simulink model "test_mdl_NI"  (R2018a)
settings: Solver=VariableStepAuto  StartTime=0.0  StopTime=10.0  RelTol=1e-3
(part 8 of 24)

== system test_mdl_NI/Subsystem/ECM_Diesel/Powertrain_Data_4_Ox424 ==
  in_port : Inport
  BpedDrvMsgTxt_B_Dsply : Terminator
  FuelLvlWarn_D_ActlEng : Terminator
  FuelLvl_Pc_DsplyEng : Terminator
  FuelRange_L_DsplyEng : Terminator
  RearDiffOilTeWarn_B_Rq : Terminator
  RearDiffOil_Te_Actl : Terminator
  SelDrvMdePt_D_Stat : Terminator
  bus_selector : BusSelector  OutputSignals=BpedDrvMsgTxt_B_Dsply,FuelLvlWarn_D_ActlEng,FuelLvl_Pc_DsplyEng,FuelRange_L_DsplyEng,RearDiffOilTeWarn_B_Rq,RearDiffOil_Te_Actl,SelDrvMdePt_D_Stat
  wires:
  in_port/1 -> bus_selector/1  "Powertrain_Data_4_Ox424"
  bus_selector/1 -> BpedDrvMsgTxt_B_Dsply/1  "<BpedDrvMsgTxt_B_Dsply>"
  bus_selector/2 -> FuelLvlWarn_D_ActlEng/1  "<FuelLvlWarn_D_ActlEng>"
  bus_selector/3 -> FuelLvl_Pc_DsplyEng/1  "<FuelLvl_Pc_DsplyEng>"
  bus_selector/4 -> FuelRange_L_DsplyEng/1  "<FuelRange_L_DsplyEng>"
  bus_selector/5 -> RearDiffOilTeWarn_B_Rq/1  "<RearDiffOilTeWarn_B_Rq>"
  bus_selector/6 -> RearDiffOil_Te_Actl/1  "<RearDiffOil_Te_Actl>"
  bus_selector/7 -> SelDrvMdePt_D_Stat/1  "<SelDrvMdePt_D_Stat>"

== system test_mdl_NI/Subsystem/ECM_Diesel/Powertrain_Data_5_Ox43F ==
  in_port : Inport
  AdasLcObtclAbrt_B_Stat : Terminator
  AirDamPos_D_Stat : Terminator
  BattRgenLoChrg_D_RqEng : Terminator
  BattRgenLoDChrg_D_RqEng : Terminator
  FapLcActv_B_Stat : Terminator
  FapLcInhbt_B_Rq : Terminator
  FapLcMaxGrdAbrt_B_Stat : Terminator
  FapLcMaxGrdInhbt_B_Stat : Terminator
  FapLcObstcl_B_Stat : Terminator
  FapLcPrchgBrk_B_Rq : Terminator
  FapLcStopHold_B_Rq : Terminator
  bus_selector : BusSelector  OutputSignals=AdasLcObtclAbrt_B_Stat,AirDamPos_D_Stat,BattRgenLoChrg_D_RqEng,BattRgenLoDChrg_D_RqEng,FapLcActv_B_Stat,FapLcInhbt_B_Rq,FapLcMaxGrdAbrt_B_Stat,FapLcMaxGrdInhbt_B_Stat,FapLcObstcl_B_Stat,FapLcPrchgBrk_B_Rq,FapLcStopHold_B_Rq
  wires:
  in_port/1 -> bus_selector/1  "Powertrain_Data_5_Ox43F"
  bus_selector/1 -> AdasLcObtclAbrt_B_Stat/1  "<AdasLcObtclAbrt_B_Stat>"
  bus_selector/2 -> AirDamPos_D_Stat/1  "<AirDamPos_D_Stat>"
  bus_selector/3 -> BattRgenLoChrg_D_RqEng/1  "<BattRgenLoChrg_D_RqEng>"
  bus_selector/4 -> BattRgenLoDChrg_D_RqEng/1  "<BattRgenLoDChrg_D_RqEng>"
  bus_selector/5 -> FapLcActv_B_Stat/1  "<FapLcActv_B_Stat>"
  bus_selector/6 -> FapLcInhbt_B_Rq/1  "<FapLcInhbt_B_Rq>"
  bus_selector/7 -> FapLcMaxGrdAbrt_B_Stat/1  "<FapLcMaxGrdAbrt_B_Stat>"
  bus_selector/8 -> FapLcMaxGrdInhbt_B_Stat/1  "<FapLcMaxGrdInhbt_B_Stat>"
  bus_selector/9 -> FapLcObstcl_B_Stat/1  "<FapLcObstcl_B_Stat>"
  bus_selector/10 -> FapLcPrchgBrk_B_Rq/1  "<FapLcPrchgBrk_B_Rq>"
  bus_selector/11 -> FapLcStopHold_B_Rq/1  "<FapLcStopHold_B_Rq>"

== system test_mdl_NI/Subsystem/ECM_Diesel/Stop_Start_Ox166 ==
  in_port : Inport
  AutoStopPtDelta_I_Est : Terminator
  HiElPwInhbt_B_Stat : Terminator
  OdoTripVerify_L_Actl : Terminator
  StopStrtDrvMde_D_Indic : Terminator
  StopStrtIODTxt_D_Rq : Terminator
  StopStrtMsgTxt_D_Rq : Terminator
  StopStrtStdby_D_Indic : Terminator
  bus_selector : BusSelector  OutputSignals=AutoStopPtDelta_I_Est,HiElPwInhbt_B_Stat,OdoTripVerify_L_Actl,StopStrtDrvMde_D_Indic,StopStrtIODTxt_D_Rq,StopStrtMsgTxt_D_Rq,StopStrtStdby_D_Indic
  wires:
  in_port/1 -> bus_selector/1  "Stop_Start_Ox166"
  bus_selector/1 -> AutoStopPtDelta_I_Est/1  "<AutoStopPtDelta_I_Est>"
  bus_selector/2 -> HiElPwInhbt_B_Stat/1  "<HiElPwInhbt_B_Stat>"
  bus_selector/3 -> OdoTripVerify_L_Actl/1  "<OdoTripVerify_L_Actl>"
  bus_selector/4 -> StopStrtDrvMde_D_Indic/1  "<StopStrtDrvMde_D_Indic>"
  bus_selector/5 -> StopStrtIODTxt_D_Rq/1  "<StopStrtIODTxt_D_Rq>"
  bus_selector/6 -> StopStrtMsgTxt_D_Rq/1  "<StopStrtMsgTxt_D_Rq>"
  bus_selector/7 -> StopStrtStdby_D_Indic/1  "<StopStrtStdby_D_Indic>"

== system test_mdl_NI/Subsystem/ECM_Diesel/TesterPhysicalResPCM_Ox7E8 ==
  in_port : Inport
  TesterPhysicalResPCM : Terminator
  bus_selector : BusSelector  OutputSignals=TesterPhysicalResPCM
  wires:
  in_port/1 -> bus_selector/1  "TesterPhysicalResPCM_Ox7E8"
  bus_selector/1 -> TesterPhysicalResPCM/1  "<TesterPhysicalResPCM>"

== system test_mdl_NI/Subsystem/ECM_Diesel/TesterPhysicalResSOBDMCFD1_Ox7EE ==
  in_port : Inport
  TesterPhysicalResSOBDMC : Terminator
  bus_selector : BusSelector  OutputSignals=TesterPhysicalResSOBDMC
  wires:
  in_port/1 -> bus_selector/1  "TesterPhysicalResSOBDMCFD1_Ox7EE"
  bus_selector/1 -> TesterPhysicalResSOBDMC/1  "<TesterPhysicalResSOBDMC>"

== system test_mdl_NI/Subsystem/ECM_Diesel/TorqueDataEngFlags_Ox200 ==
  in_port : Inport
  PrplWhlTotTqRq_No_Cnt : Terminator
  PrplWhlTotTqRq_No_Cs : Terminator
  PrplWhlTot_Tq_LimMn : Terminator
  PrplWhlTot_Tq_Rq : Terminator
  PtDrvMde_D_Stat : Terminator
  bus_selector : BusSelector  OutputSignals=PrplWhlTotTqRq_No_Cnt,PrplWhlTotTqRq_No_Cs,PrplWhlTot_Tq_LimMn,PrplWhlTot_Tq_Rq,PtDrvMde_D_Stat
  wires:
  in_port/1 -> bus_selector/1  "TorqueDataEngFlags_Ox200"
  bus_selector/1 -> PrplWhlTotTqRq_No_Cnt/1  "<PrplWhlTotTqRq_No_Cnt>"
  bus_selector/2 -> PrplWhlTotTqRq_No_Cs/1  "<PrplWhlTotTqRq_No_Cs>"
  bus_selector/3 -> PrplWhlTot_Tq_LimMn/1  "<PrplWhlTot_Tq_LimMn>"
  bus_selector/4 -> PrplWhlTot_Tq_Rq/1  "<PrplWhlTot_Tq_Rq>"
  bus_selector/5 -> PtDrvMde_D_Stat/1  "<PtDrvMde_D_Stat>"

== system test_mdl_NI/Subsystem/ECM_Diesel/VehicleOperatingModes_Ox167 ==
  in_port : Inport
  ElPw_D_Stat : Terminator
  ElPw_D_StatStrtStop : Terminator
  Eng_D_Stat : Terminator
  PlgActvArb_B_Actl : Terminator
  PrplWhlRgenMn_Tq_Actl : Terminator
  PrplWhlTot2_Tq_Actl : Terminator
  PwPckTq_D_Stat : Terminator
  TrnAinTq_D_Qf : Terminator
  TrnAin_Tq_Actl : Terminator
  bus_selector : BusSelector  OutputSignals=ElPw_D_Stat,ElPw_D_StatStrtStop,Eng_D_Stat,PlgActvArb_B_Actl,PrplWhlRgenMn_Tq_Actl,PrplWhlTot2_Tq_Actl,PwPckTq_D_Stat,TrnAinTq_D_Qf,TrnAin_Tq_Actl
  wires:
  in_port/1 -> bus_selector/1  "VehicleOperatingModes_Ox167"
  bus_selector/1 -> ElPw_D_Stat/1  "<ElPw_D_Stat>"
  bus_selector/2 -> ElPw_D_StatStrtStop/1  "<ElPw_D_StatStrtStop>"
  bus_selector/3 -> Eng_D_Stat/1  "<Eng_D_Stat>"
  bus_selector/4 -> PlgActvArb_B_Actl/1  "<PlgActvArb_B_Actl>"
  bus_selector/5 -> PrplWhlRgenMn_Tq_Actl/1  "<PrplWhlRgenMn_Tq_Actl>"
  bus_selector/6 -> PrplWhlTot2_Tq_Actl/1  "<PrplWhlTot2_Tq_Actl>"
  bus_selector/7 -> PwPckTq_D_Stat/1  "<PwPckTq_D_Stat>"
  bus_selector/8 -> TrnAinTq_D_Qf/1  "<TrnAinTq_D_Qf>"
  bus_selector/9 -> TrnAin_Tq_Actl/1  "<TrnAin_Tq_Actl>"

== system test_mdl_NI/Subsystem/GWM/AC_Compressor_Data_FD1_Ox411 ==
  in_port : Inport
  ElCmprBattSysU_D_Falt : Terminator
  ElCmprBattURng_D_Falt : Terminator
  ElCmprInnrErr_D_Falt : Terminator
  ElCmprLostComm_D_Falt : Terminator
  ElCmprOverLoad_D_Falt : Terminator
  ElCmprOverTe_D_Falt : Terminator
  ElCmprOverTe_D_Stat : Terminator
  ElCmprPerfErr_D_Falt : Terminator
  ElCmprSysU_D_Falt : Terminator
  ElCmprUHi_D_Stat : Terminator
  ElCmprUHi_U_Actl : Terminator
  ElCmpr_D_Stat : Terminator
  ElCmpr_N_Actl : Terminator
  ElCmpr_Pw_Actl : Terminator
  bus_selector : BusSelector  OutputSignals=ElCmprBattSysU_D_Falt,ElCmprBattURng_D_Falt,ElCmprInnrErr_D_Falt,ElCmprLostComm_D_Falt,ElCmprOverLoad_D_Falt,ElCmprOverTe_D_Falt,ElCmprOverTe_D_Stat,ElCmprPerfErr_D_Falt,ElCmprSysU_D_Falt,ElCmprUHi_D_Stat,ElCmprUHi_U_Actl,ElCmpr_D_Stat,ElCmpr_N_Actl,ElCmpr_Pw_Actl
  wires:
  in_port/1 -> bus_selector/1  "AC_Compressor_Data_FD1_Ox411"
  bus_selector/1 -> ElCmprBattSysU_D_Falt/1  "<ElCmprBattSysU_D_Falt>"
  bus_selector/2 -> ElCmprBattURng_D_Falt/1  "<ElCmprBattURng_D_Falt>"
  bus_selector/3 -> ElCmprInnrErr_D_Falt/1  "<ElCmprInnrErr_D_Falt>"
  bus_selector/4 -> ElCmprLostComm_D_Falt/1  "<ElCmprLostComm_D_Falt>"
  bus_selector/5 -> ElCmprOverLoad_D_Falt/1  "<ElCmprOverLoad_D_Falt>"
  bus_selector/6 -> ElCmprOverTe_D_Falt/1  "<ElCmprOverTe_D_Falt>"
  bus_selector/7 -> ElCmprOverTe_D_Stat/1  "<ElCmprOverTe_D_Stat>"
  bus_selector/8 -> ElCmprPerfErr_D_Falt/1  "<ElCmprPerfErr_D_Falt>"
  bus_selector/9 -> ElCmprSysU_D_Falt/1  "<ElCmprSysU_D_Falt>"
  bus_selector/10 -> ElCmprUHi_D_Stat/1  "<ElCmprUHi_D_Stat>"
  bus_selector/11 -> ElCmprUHi_U_Actl/1  "<ElCmprUHi_U_Actl>"
  bus_selector/12 -> ElCmpr_D_Stat/1  "<ElCmpr_D_Stat>"
  bus_selector/13 -> ElCmpr_N_Actl/1  "<ElCmpr_N_Actl>"
  bus_selector/14 -> ElCmpr_Pw_Actl/1  "<ElCmpr_Pw_Actl>"

== system test_mdl_NI/Subsystem/GWM/APIMGPS_Data_Nav_1_FD1_Ox462 ==
  in_port : Inport
  GPS_Latitude_Degrees : Terminator
  GPS_Latitude_Min_dec : Terminator
  GPS_Latitude_Minutes : Terminator
  GPS_Longitude_Degrees : Terminator
  GPS_Longitude_Min_dec : Terminator
  GPS_Longitude_Minutes : Terminator
  GpsHsphLattSth_D_Actl : Terminator
  GpsHsphLongEast_D_Actl : Terminator
  bus_selector : BusSelector  OutputSignals=GPS_Latitude_Degrees,GPS_Latitude_Min_dec,GPS_Latitude_Minutes,GPS_Longitude_Degrees,GPS_Longitude_Min_dec,GPS_Longitude_Minutes,GpsHsphLattSth_D_Actl,GpsHsphLongEast_D_Actl
  wires:
  in_port/1 -> bus_selector/1  "APIMGPS_Data_Nav_1_FD1_Ox462"
  bus_selector/1 -> GPS_Latitude_Degrees/1  "<GPS_Latitude_Degrees>"
  bus_selector/2 -> GPS_Latitude_Min_dec/1  "<GPS_Latitude_Min_dec>"
  bus_selector/3 -> GPS_Latitude_Minutes/1  "<GPS_Latitude_Minutes>"
  bus_selector/4 -> GPS_Longitude_Degrees/1  "<GPS_Longitude_Degrees>"
  bus_selector/5 -> GPS_Longitude_Min_dec/1  "<GPS_Longitude_Min_dec>"
  bus_selector/6 -> GPS_Longitude_Minutes/1  "<GPS_Longitude_Minutes>"
  bus_selector/7 -> GpsHsphLattSth_D_Actl/1  "<GpsHsphLattSth_D_Actl>"
  bus_selector/8 -> GpsHsphLongEast_D_Actl/1  "<GpsHsphLongEast_D_Actl>"

== system test_mdl_NI/Subsystem/GWM/APIMGPS_Data_Nav_2_FD1_Ox463 ==
  in_port : Inport
  GPS_Actual_vs_Infer_pos : Terminator
  GPS_Compass_direction : Terminator
  GPS_Pdop : Terminator
  GPS_UTC_hours : Terminator
  GPS_UTC_minutes : Terminator
  GPS_UTC_seconds : Terminator
  GpsUtcDay_No_Actl : Terminator
  GpsUtcMnth_No_Actl : Terminator
  GpsUtcYr_No_Actl : Terminator
  Gps_B_Falt : Terminator
  bus_selector : BusSelector  OutputSignals=GPS_Actual_vs_Infer_pos,GPS_Compass_direction,GPS_Pdop,GPS_UTC_hours,GPS_UTC_minutes,GPS_UTC_seconds,GpsUtcDay_No_Actl,GpsUtcMnth_No_Actl,GpsUtcYr_No_Actl,Gps_B_Falt
  wires:
  in_port/1 -> bus_selector/1  "APIMGPS_Data_Nav_2_FD1_Ox463"
  bus_selector/1 -> GPS_Actual_vs_Infer_pos/1  "<GPS_Actual_vs_Infer_pos>"
  bus_selector/2 -> GPS_Compass_direction/1  "<GPS_Compass_direction>"
  bus_selector/3 -> GPS_Pdop/1  "<GPS_Pdop>"
  bus_selector/4 -> GPS_UTC_hours/1  "<GPS_UTC_hours>"
  bus_selector/5 -> GPS_UTC_minutes/1  "<GPS_UTC_minutes>"
  bus_selector/6 -> GPS_UTC_seconds/1  "<GPS_UTC_seconds>"
  bus_selector/7 -> GpsUtcDay_No_Actl/1  "<GpsUtcDay_No_Actl>"
  bus_selector/8 -> GpsUtcMnth_No_Actl/1  "<GpsUtcMnth_No_Actl>"
  bus_selector/9 -> GpsUtcYr_No_Actl/1  "<GpsUtcYr_No_Actl>"
  bus_selector/10 -> Gps_B_Falt/1  "<Gps_B_Falt>"

== system test_mdl_NI/Subsystem/GWM/APIMGPS_Data_Nav_3_FD1_Ox464 ==
  in_port : Inport
  GPS_Hdop : Terminator
  GPS_Heading : Terminator
  GPS_MSL_altitude : Terminator
  GPS_Sat_num_in_view : Terminator
  GPS_Speed : Terminator
  GPS_Vdop : Terminator
  GPS_dimension : Terminator
  bus_selector : BusSelector  OutputSignals=GPS_Hdop,GPS_Heading,GPS_MSL_altitude,GPS_Sat_num_in_view,GPS_Speed,GPS_Vdop,GPS_dimension
  wires:
  in_port/1 -> bus_selector/1  "APIMGPS_Data_Nav_3_FD1_Ox464"
  bus_selector/1 -> GPS_Hdop/1  "<GPS_Hdop>"
  bus_selector/2 -> GPS_Heading/1  "<GPS_Heading>"
  bus_selector/3 -> GPS_MSL_altitude/1  "<GPS_MSL_altitude>"
  bus_selector/4 -> GPS_Sat_num_in_view/1  "<GPS_Sat_num_in_view>"
  bus_selector/5 -> GPS_Speed/1  "<GPS_Speed>"
  bus_selector/6 -> GPS_Vdop/1  "<GPS_Vdop>"
  bus_selector/7 -> GPS_dimension/1  "<GPS_dimension>"

== system test_mdl_NI/Subsystem/GWM/APIM_Data_FD1_Ox32B ==
  in_port : Inport
  AutoLghtOvrrd_B_RqDrv : Terminator
  DistToStopover_L_Actl : Terminator
  ExtLghtDsply_D_Stat : Terminator
  ExtLghtFront_D_RqMnu : Terminator
  ExtLghtLeft_D_RqMnu : Terminator
  ExtLghtRear_D_RqMnu : Terminator
  ExtLghtRight_D_RqMnu : Terminator
  GoTEditHr_T_RqMnu : Terminator
  GoTEditMnte_T_RqMnu : Terminator
  StopoverType_D_Stat : Terminator
  bus_selector : BusSelector  OutputSignals=AutoLghtOvrrd_B_RqDrv,DistToStopover_L_Actl,ExtLghtDsply_D_Stat,ExtLghtFront_D_RqMnu,ExtLghtLeft_D_RqMnu,ExtLghtRear_D_RqMnu,ExtLghtRight_D_RqMnu,GoTEditHr_T_RqMnu,GoTEditMnte_T_RqMnu,StopoverType_D_Stat
  wires:
  in_port/1 -> bus_selector/1  "APIM_Data_FD1_Ox32B"
  bus_selector/1 -> AutoLghtOvrrd_B_RqDrv/1  "<AutoLghtOvrrd_B_RqDrv>"
  bus_selector/2 -> DistToStopover_L_Actl/1  "<DistToStopover_L_Actl>"
  bus_selector/3 -> ExtLghtDsply_D_Stat/1  "<ExtLghtDsply_D_Stat>"
  bus_selector/4 -> ExtLghtFront_D_RqMnu/1  "<ExtLghtFront_D_RqMnu>"
  bus_selector/5 -> ExtLghtLeft_D_RqMnu/1  "<ExtLghtLeft_D_RqMnu>"
  bus_selector/6 -> ExtLghtRear_D_RqMnu/1  "<ExtLghtRear_D_RqMnu>"
  bus_selector/7 -> ExtLghtRight_D_RqMnu/1  "<ExtLghtRight_D_RqMnu>"
  bus_selector/8 -> GoTEditHr_T_RqMnu/1  "<GoTEditHr_T_RqMnu>"
  bus_selector/9 -> GoTEditMnte_T_RqMnu/1  "<GoTEditMnte_T_RqMnu>"
  bus_selector/10 -> StopoverType_D_Stat/1  "<StopoverType_D_Stat>"

== system test_mdl_NI/Subsystem/GWM/APIM_Request_Signals_1_FD1_Ox227 ==
  in_port : Inport
  Btt_L_Actl2 : Terminator
  ChrgCrdLckEnbl_B_Stat : Terminator
  ChrgOvrdExitScrn_D_Rq : Terminator
  Cntr_Plg_Mode_Cmd : Terminator
  EmPrflButtnAssoc_D_Rq : Terminator
  EmPrflKeyAssoc_D_Rq : Terminator
  EmPrflNo_D_Rq : Terminator
  Em_D_Stat : Terminator
  PmCabnLvl_D_Stat : Terminator
  PmCabn_D_Stat : Terminator
  PwRnngBoardMde_D_Rq : Terminator
  PwRnngBoardSwtch_D_Rq : Terminator
  PwRnngBoardT_D_Rq : Terminator
  Rba_D_Rq : Terminator
  bus_selector : BusSelector  OutputSignals=Btt_L_Actl2,ChrgCrdLckEnbl_B_Stat,ChrgOvrdExitScrn_D_Rq,Cntr_Plg_Mode_Cmd,EmPrflButtnAssoc_D_Rq,EmPrflKeyAssoc_D_Rq,EmPrflNo_D_Rq,Em_D_Stat,PmCabnLvl_D_Stat,PmCabn_D_Stat,PwRnngBoardMde_D_Rq,PwRnngBoardSwtch_D_Rq,PwRnngBoardT_D_Rq,Rba_D_Rq
  wires:
  in_port/1 -> bus_selector/1  "APIM_Request_Signals_1_FD1_Ox227"
  bus_selector/1 -> Btt_L_Actl2/1  "<Btt_L_Actl2>"
  bus_selector/2 -> ChrgCrdLckEnbl_B_Stat/1  "<ChrgCrdLckEnbl_B_Stat>"
  bus_selector/3 -> ChrgOvrdExitScrn_D_Rq/1  "<ChrgOvrdExitScrn_D_Rq>"
  bus_selector/4 -> Cntr_Plg_Mode_Cmd/1  "<Cntr_Plg_Mode_Cmd>"
  bus_selector/5 -> EmPrflButtnAssoc_D_Rq/1  "<EmPrflButtnAssoc_D_Rq>"
  bus_selector/6 -> EmPrflKeyAssoc_D_Rq/1  "<EmPrflKeyAssoc_D_Rq>"
  bus_selector/7 -> EmPrflNo_D_Rq/1  "<EmPrflNo_D_Rq>"
  bus_selector/8 -> Em_D_Stat/1  "<Em_D_Stat>"
  bus_selector/9 -> PmCabnLvl_D_Stat/1  "<PmCabnLvl_D_Stat>"
  bus_selector/10 -> PmCabn_D_Stat/1  "<PmCabn_D_Stat>"
  bus_selector/11 -> PwRnngBoardMde_D_Rq/1  "<PwRnngBoardMde_D_Rq>"
  bus_selector/12 -> PwRnngBoardSwtch_D_Rq/1  "<PwRnngBoardSwtch_D_Rq>"
  bus_selector/13 -> PwRnngBoardT_D_Rq/1  "<PwRnngBoardT_D_Rq>"
  bus_selector/14 -> Rba_D_Rq/1  "<Rba_D_Rq>"

== system test_mdl_NI/Subsystem/GWM/APIM_Request_Signals_5_FD1_Ox211 ==
  in_port : Inport
  OnbChrgLocIdTrgt_No_Rq : Terminator
  OnbChrgLocIdUns_B_Rq : Terminator
  OnbChrgPrflUpdate_B_Rq : Terminator
  OnbChrgPrflWkdy_No_Rq : Terminator
  OnbChrgPrflWknd_No_Rq : Terminator
  OnbChrgSetDelete_B_Rq : Terminator
  OnbChrgSetNow_D_Rq : Terminator
  OnbChrgToPcWkdy_D_Actl : Terminator
  OnbChrgToPcWknd_D_Actl : Terminator
  bus_selector : BusSelector  OutputSignals=OnbChrgLocIdTrgt_No_Rq,OnbChrgLocIdUns_B_Rq,OnbChrgPrflUpdate_B_Rq,OnbChrgPrflWkdy_No_Rq,OnbChrgPrflWknd_No_Rq,OnbChrgSetDelete_B_Rq,OnbChrgSetNow_D_Rq,OnbChrgToPcWkdy_D_Actl,OnbChrgToPcWknd_D_Actl
  wires:
  in_port/1 -> bus_selector/1  "APIM_Request_Signals_5_FD1_Ox211"
  bus_selector/1 -> OnbChrgLocIdTrgt_No_Rq/1  "<OnbChrgLocIdTrgt_No_Rq>"
  bus_selector/2 -> OnbChrgLocIdUns_B_Rq/1  "<OnbChrgLocIdUns_B_Rq>"
  bus_selector/3 -> OnbChrgPrflUpdate_B_Rq/1  "<OnbChrgPrflUpdate_B_Rq>"
  bus_selector/4 -> OnbChrgPrflWkdy_No_Rq/1  "<OnbChrgPrflWkdy_No_Rq>"
  bus_selector/5 -> OnbChrgPrflWknd_No_Rq/1  "<OnbChrgPrflWknd_No_Rq>"
  bus_selector/6 -> OnbChrgSetDelete_B_Rq/1  "<OnbChrgSetDelete_B_Rq>"
  bus_selector/7 -> OnbChrgSetNow_D_Rq/1  "<OnbChrgSetNow_D_Rq>"
  bus_selector/8 -> OnbChrgToPcWkdy_D_Actl/1  "<OnbChrgToPcWkdy_D_Actl>"
  bus_selector/9 -> OnbChrgToPcWknd_D_Actl/1  "<OnbChrgToPcWknd_D_Actl>"

== system test_mdl_NI/Subsystem/GWM/APIM_Request_Signals_FD1_Ox105 ==
  in_port : Inport
  CbnCmrtPrefListIndx_Rq : Terminator
  CbnCmrtPrefLstNmItm_Rq : Terminator
  ChrgStatDsply_D_Rq : Terminator
  FactoryReset_Rq : Terminator
  LongTermParking_Rq : Terminator
  ModemReset_D_Rq : Terminator
  NextUsageTimeToggle_Rq : Terminator
  OffPeakTimeSetHR_Rq : Terminator
  OffPeakTimeSetMin_Rq : Terminator
  StopStrtDrvMde_B_RqBtn3 : Terminator
  TCU_ESN_D_Rq : Terminator
  bus_selector : BusSelector  OutputSignals=CbnCmrtPrefListIndx_Rq,CbnCmrtPrefLstNmItm_Rq,ChrgStatDsply_D_Rq,FactoryReset_Rq,LongTermParking_Rq,ModemReset_D_Rq,NextUsageTimeToggle_Rq,OffPeakTimeSetHR_Rq,OffPeakTimeSetMin_Rq,StopStrtDrvMde_B_RqBtn3,TCU_ESN_D_Rq
  wires:
  in_port/1 -> bus_selector/1  "APIM_Request_Signals_FD1_Ox105"
  bus_selector/1 -> CbnCmrtPrefListIndx_Rq/1  "<CbnCmrtPrefListIndx_Rq>"
  bus_selector/2 -> CbnCmrtPrefLstNmItm_Rq/1  "<CbnCmrtPrefLstNmItm_Rq>"
  bus_selector/3 -> ChrgStatDsply_D_Rq/1  "<ChrgStatDsply_D_Rq>"
  bus_selector/4 -> FactoryReset_Rq/1  "<FactoryReset_Rq>"
  bus_selector/5 -> LongTermParking_Rq/1  "<LongTermParking_Rq>"
  bus_selector/6 -> ModemReset_D_Rq/1  "<ModemReset_D_Rq>"
  bus_selector/7 -> NextUsageTimeToggle_Rq/1  "<NextUsageTimeToggle_Rq>"
  bus_selector/8 -> OffPeakTimeSetHR_Rq/1  "<OffPeakTimeSetHR_Rq>"
  bus_selector/9 -> OffPeakTimeSetMin_Rq/1  "<OffPeakTimeSetMin_Rq>"
  bus_selector/10 -> StopStrtDrvMde_B_RqBtn3/1  "<StopStrtDrvMde_B_RqBtn3>"
  bus_selector/11 -> TCU_ESN_D_Rq/1  "<TCU_ESN_D_Rq>"

== system test_mdl_NI/Subsystem/GWM/APIM_Send_Signals1_FD1_Ox3F1 ==
  in_port : Inport
  APIM_ActiveTrackNum_St : Terminator
  APIM_NumberofTracks_St : Terminator
  AutoHoldSwtch_D_Stat3 : Terminator
  CenterStackRing_D_Actl : Terminator
  ChrgCordUnlock_B_Rq : Terminator
  TrlrAidCancl_B_Rq : Terminator
  TrlrAidSetup_D_Stat : Terminator
  TrlrTrgtAcquire_D_Rq : Terminator
  ValetMode_D_Stat : Terminator
  bus_selector : BusSelector  OutputSignals=APIM_ActiveTrackNum_St,APIM_NumberofTracks_St,AutoHoldSwtch_D_Stat3,CenterStackRing_D_Actl,ChrgCordUnlock_B_Rq,TrlrAidCancl_B_Rq,TrlrAidSetup_D_Stat,TrlrTrgtAcquire_D_Rq,ValetMode_D_Stat
  wires:
  in_port/1 -> bus_selector/1  "APIM_Send_Signals1_FD1_Ox3F1"
  bus_selector/1 -> APIM_ActiveTrackNum_St/1  "<APIM_ActiveTrackNum_St>"
  bus_selector/2 -> APIM_NumberofTracks_St/1  "<APIM_NumberofTracks_St>"
  bus_selector/3 -> AutoHoldSwtch_D_Stat3/1  "<AutoHoldSwtch_D_Stat3>"
  bus_selector/4 -> CenterStackRing_D_Actl/1  "<CenterStackRing_D_Actl>"
  bus_selector/5 -> ChrgCordUnlock_B_Rq/1  "<ChrgCordUnlock_B_Rq>"
  bus_selector/6 -> TrlrAidCancl_B_Rq/1  "<TrlrAidCancl_B_Rq>"
  bus_selector/7 -> TrlrAidSetup_D_Stat/1  "<TrlrAidSetup_D_Stat>"
  bus_selector/8 -> TrlrTrgtAcquire_D_Rq/1  "<TrlrTrgtAcquire_D_Rq>"
  bus_selector/9 -> ValetMode_D_Stat/1  "<ValetMode_D_Stat>"

== system test_mdl_NI/Subsystem/GWM/APIM_Send_Signals_2_FD1_Ox215 ==
  in_port : Inport
  AutoEpbButtn_B_Stat : Terminator
  AutoEpbZoomView_B_Stat : Terminator
  DcacGfciTestBttn_B_Stat : Terminator
  DcacPwButtn_B_Falt : Terminator
  DcacPwHiButtn_B_Stat : Terminator
  DcacPwLoButtn_B_Stat : Terminator
  DcacPwOffButtn_B_Stat : Terminator
  DcacPwResetButtn_B_Stat : Terminator
  OnbChrgClearAll_B_Rq : Terminator
  OnbChrgGoTDelete_B_Rq : Terminator
  OnbChrgGoTElement_D_Rq : Terminator
  OnbChrgGoTExtHtr_D_Rq : Terminator
  OnbChrgGoTHr_T_Rq : Terminator
  OnbChrgGoTMnte_D_Rq : Terminator
  OnbChrgGoTOn_D_Rq : Terminator
  OnbChrgGoTPrcond_D_Rq : Terminator
  OnbChrgGoTTouch_D_Rq : Terminator
  OnbChrgGoTUpdate_B_Rq : Terminator
  OtaTrg_D_Stat : Terminator
  PaakMyKey_D_Rq : Terminator
  TCU_Final_Actvtn_St : Terminator
  TCU_Init_Actvtn_St : Terminator
  TrlrAidMde_D_Rq : Terminator
  TrlrBrkGain_No_Rq : Terminator
  TrlrHitch_D_RqMnu : Terminator
  bus_selector : BusSelector  OutputSignals=AutoEpbButtn_B_Stat,AutoEpbZoomView_B_Stat,DcacGfciTestBttn_B_Stat,DcacPwButtn_B_Falt,DcacPwHiButtn_B_Stat,DcacPwLoButtn_B_Stat,DcacPwOffButtn_B_Stat,DcacPwResetButtn_B_Stat,OnbChrgClearAll_B_Rq,OnbChrgGoTDelete_B_Rq,OnbChrgGoTElement_D_Rq,OnbChrgGoTExtHtr_D_Rq,OnbChrgGoTHr_T_Rq,OnbChrgGoTMnte_D_Rq,OnbChrgGoTOn_D_Rq,OnbChrgGoTPrcond_D_Rq,OnbChrgGoTTouch_D_Rq,OnbChrgGoTUpdate_B_Rq,OtaTrg_D_Stat,PaakMyKey_D_Rq,TCU_Final_Actvtn_St,TCU_Init_Actvtn_St,TrlrAidMde_D_Rq,TrlrBrkGain_No_Rq,TrlrHitch_D_RqMnu
  wires:
  in_port/1 -> bus_selector/1  "APIM_Send_Signals_2_FD1_Ox215"
  bus_selector/1 -> AutoEpbButtn_B_Stat/1  "<AutoEpbButtn_B_Stat>"
  bus_selector/2 -> AutoEpbZoomView_B_Stat/1  "<AutoEpbZoomView_B_Stat>"
  bus_selector/3 -> DcacGfciTestBttn_B_Stat/1  "<DcacGfciTestBttn_B_Stat>"
  bus_selector/4 -> DcacPwButtn_B_Falt/1  "<DcacPwButtn_B_Falt>"
  bus_selector/5 -> DcacPwHiButtn_B_Stat/1  "<DcacPwHiButtn_B_Stat>"
  bus_selector/6 -> DcacPwLoButtn_B_Stat/1  "<DcacPwLoButtn_B_Stat>"
  bus_selector/7 -> DcacPwOffButtn_B_Stat/1  "<DcacPwOffButtn_B_Stat>"
  bus_selector/8 -> DcacPwResetButtn_B_Stat/1  "<DcacPwResetButtn_B_Stat>"
  bus_selector/9 -> OnbChrgClearAll_B_Rq/1  "<OnbChrgClearAll_B_Rq>"
  bus_selector/10 -> OnbChrgGoTDelete_B_Rq/1  "<OnbChrgGoTDelete_B_Rq>"
  bus_selector/11 -> OnbChrgGoTElement_D_Rq/1  "<OnbChrgGoTElement_D_Rq>"
  bus_selector/12 -> OnbChrgGoTExtHtr_D_Rq/1  "<OnbChrgGoTExtHtr_D_Rq>"
  bus_selector/13 -> OnbChrgGoTHr_T_Rq/1  "<OnbChrgGoTHr_T_Rq>"
  bus_selector/14 -> OnbChrgGoTMnte_D_Rq/1  "<OnbChrgGoTMnte_D_Rq>"
  bus_selector/15 -> OnbChrgGoTOn_D_Rq/1  "<OnbChrgGoTOn_D_Rq>"
  bus_selector/16 -> OnbChrgGoTPrcond_D_Rq/1  "<OnbChrgGoTPrcond_D_Rq>"
  bus_selector/17 -> OnbChrgGoTTouch_D_Rq/1  "<OnbChrgGoTTouch_D_Rq>"
  bus_selector/18 -> OnbChrgGoTUpdate_B_Rq/1  "<OnbChrgGoTUpdate_B_Rq>"
  bus_selector/19 -> OtaTrg_D_Stat/1  "<OtaTrg_D_Stat>"
  bus_selector/20 -> PaakMyKey_D_Rq/1  "<PaakMyKey_D_Rq>"
  bus_selector/21 -> TCU_Final_Actvtn_St/1  "<TCU_Final_Actvtn_St>"
  bus_selector/22 -> TCU_Init_Actvtn_St/1  "<TCU_Init_Actvtn_St>"
  bus_selector/23 -> TrlrAidMde_D_Rq/1  "<TrlrAidMde_D_Rq>"
  bus_selector/24 -> TrlrBrkGain_No_Rq/1  "<TrlrBrkGain_No_Rq>"
  bus_selector/25 -> TrlrHitch_D_RqMnu/1  "<TrlrHitch_D_RqMnu>"

== system test_mdl_NI/Subsystem/GWM/Accel_Data_FD1_Ox92 ==
  in_port : Inport
  VehLat2_A_Actl : Terminator
  VehLatAActl_D_Qf : Terminator
  VehLatLongVertA_No_Cs : Terminator
  VehLatLongVert_No_Cnt : Terminator
  VehLong2_A_Actl : Terminator
  VehLongAActl_D_Qf : Terminator
  VehVert2_A_Actl : Terminator
  VehVertAActl_D_Qf : Terminator
  bus_selector : BusSelector  OutputSignals=VehLat2_A_Actl,VehLatAActl_D_Qf,VehLatLongVertA_No_Cs,VehLatLongVert_No_Cnt,VehLong2_A_Actl,VehLongAActl_D_Qf,VehVert2_A_Actl,VehVertAActl_D_Qf
  wires:
  in_port/1 -> bus_selector/1  "Accel_Data_FD1_Ox92"
  bus_selector/1 -> VehLat2_A_Actl/1  "<VehLat2_A_Actl>"
  bus_selector/2 -> VehLatAActl_D_Qf/1  "<VehLatAActl_D_Qf>"
  bus_selector/3 -> VehLatLongVertA_No_Cs/1  "<VehLatLongVertA_No_Cs>"
  bus_selector/4 -> VehLatLongVert_No_Cnt/1  "<VehLatLongVert_No_Cnt>"
  bus_selector/5 -> VehLong2_A_Actl/1  "<VehLong2_A_Actl>"
  bus_selector/6 -> VehLongAActl_D_Qf/1  "<VehLongAActl_D_Qf>"
  bus_selector/7 -> VehVert2_A_Actl/1  "<VehVert2_A_Actl>"
  bus_selector/8 -> VehVertAActl_D_Qf/1  "<VehVertAActl_D_Qf>"

== system test_mdl_NI/Subsystem/GWM/ActiveFrontStrg_Stat2_FD1_Ox8A ==
  in_port : Inport
  SteWhlRelCalib_An_Sns : Terminator
  SteWhlRelCalib_T_Actl : Terminator
  bus_selector : BusSelector  OutputSignals=SteWhlRelCalib_An_Sns,SteWhlRelCalib_T_Actl
  wires:
  in_port/1 -> bus_selector/1  "ActiveFrontStrg_Stat2_FD1_Ox8A"
  bus_selector/1 -> SteWhlRelCalib_An_Sns/1  "<SteWhlRelCalib_An_Sns>"
  bus_selector/2 -> SteWhlRelCalib_T_Actl/1  "<SteWhlRelCalib_T_Actl>"

== system test_mdl_NI/Subsystem/GWM/ActiveFrontStrg_Stat_FD1_Ox89 ==
  in_port : Inport
  SteWhlBrkAnActl_No_Cnt : Terminator
  SteWhlBrkAnActl_No_Cs : Terminator
  SteWhlBrkOffst_An_Actl : Terminator
  SteWhlOffstRq_D_Stat : Terminator
  SteWhlOffst_An_TotActl : Terminator
  bus_selector : BusSelector  OutputSignals=SteWhlBrkAnActl_No_Cnt,SteWhlBrkAnActl_No_Cs,SteWhlBrkOffst_An_Actl,SteWhlOffstRq_D_Stat,SteWhlOffst_An_TotActl
  wires:
  in_port/1 -> bus_selector/1  "ActiveFrontStrg_Stat_FD1_Ox89"
  bus_selector/1 -> SteWhlBrkAnActl_No_Cnt/1  "<SteWhlBrkAnActl_No_Cnt>"
  bus_selector/2 -> SteWhlBrkAnActl_No_Cs/1  "<SteWhlBrkAnActl_No_Cs>"
  bus_selector/3 -> SteWhlBrkOffst_An_Actl/1  "<SteWhlBrkOffst_An_Actl>"
  bus_selector/4 -> SteWhlOffstRq_D_Stat/1  "<SteWhlOffstRq_D_Stat>"
  bus_selector/5 -> SteWhlOffst_An_TotActl/1  "<SteWhlOffst_An_TotActl>"

== system test_mdl_NI/Subsystem/GWM/Adaptive_Headlamp_Stat_Ox334 ==
  in_port : Inport
  Adaptive_Hdlmp_Fault : Terminator
  AhbStatGfhbFdbk_D_Actl : Terminator
  HeadLghtDrvSide_B_Stat : Terminator
  HeadLghtHiOn_B_StatHcm : Terminator
  bus_selector : BusSelector  OutputSignals=Adaptive_Hdlmp_Fault,AhbStatGfhbFdbk_D_Actl,HeadLghtDrvSide_B_Stat,HeadLghtHiOn_B_StatHcm
  wires:
  in_port/1 -> bus_selector/1  "Adaptive_Headlamp_Stat_Ox334"
  bus_selector/1 -> Adaptive_Hdlmp_Fault/1  "<Adaptive_Hdlmp_Fault>"
  bus_selector/2 -> AhbStatGfhbFdbk_D_Actl/1  "<AhbStatGfhbFdbk_D_Actl>"
  bus_selector/3 -> HeadLghtDrvSide_B_Stat/1  "<HeadLghtDrvSide_B_Stat>"
  bus_selector/4 -> HeadLghtHiOn_B_StatHcm/1  "<HeadLghtHiOn_B_StatHcm>"

== system test_mdl_NI/Subsystem/GWM/AllTerrainControlData_FD1_Ox461 ==
  in_port : Inport
  SelDrvMdeCnt_D_Stat : Terminator
  SelDrvMdeSwtch_D_Stat : Terminator
  SelDrvMdeSwtch_No_Actl : Terminator
  bus_selector : BusSelector  OutputSignals=SelDrvMdeCnt_D_Stat,SelDrvMdeSwtch_D_Stat,SelDrvMdeSwtch_No_Actl
  wires:
  in_port/1 -> bus_selector/1  "AllTerrainControlData_FD1_Ox461"
  bus_selector/1 -> SelDrvMdeCnt_D_Stat/1  "<SelDrvMdeCnt_D_Stat>"
  bus_selector/2 -> SelDrvMdeSwtch_D_Stat/1  "<SelDrvMdeSwtch_D_Stat>"
  bus_selector/3 -> SelDrvMdeSwtch_No_Actl/1  "<SelDrvMdeSwtch_No_Actl>"

== system test_mdl_NI/Subsystem/GWM/All_Terrain_Data_FD1_Ox481 ==
  in_port : Inport
  TerrMde_D_RqDrv : Terminator
  bus_selector : BusSelector  OutputSignals=TerrMde_D_RqDrv
  wires:
  in_port/1 -> bus_selector/1  "All_Terrain_Data_FD1_Ox481"
  bus_selector/1 -> TerrMde_D_RqDrv/1  "<TerrMde_D_RqDrv>"

== system test_mdl_NI/Subsystem/GWM/BCMC_Data_FD1_Ox36F ==
  in_port : Inport
  WndwRearHeat_D_Stat : Terminator
  WndwRearHeat_I_Actl : Terminator
  bus_selector : BusSelector  OutputSignals=WndwRearHeat_D_Stat,WndwRearHeat_I_Actl
  wires:
  in_port/1 -> bus_selector/1  "BCMC_Data_FD1_Ox36F"
  bus_selector/1 -> WndwRearHeat_D_Stat/1  "<WndwRearHeat_D_Stat>"
  bus_selector/2 -> WndwRearHeat_I_Actl/1  "<WndwRearHeat_I_Actl>"

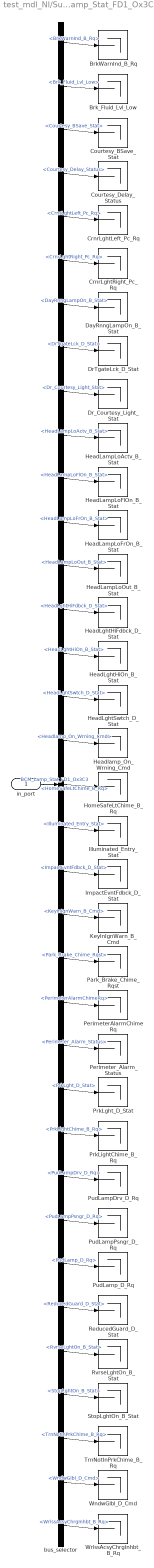
== system test_mdl_NI/Subsystem/GWM/BCM_Lamp_Stat_FD1_Ox3C3 ==
  in_port : Inport
  BrkWarnInd_B_Rq : Terminator
  Brk_Fluid_Lvl_Low : Terminator
  Courtesy_BSave_Stat : Terminator
  Courtesy_Delay_Status : Terminator
  CrnrLghtLeft_Pc_Rq : Terminator
  CrnrLghtRight_Pc_Rq : Terminator
  DayRnngLampOn_B_Stat : Terminator
  DrTgateLck_D_Stat : Terminator
  Dr_Courtesy_Light_Stat : Terminator
  HeadLampLoActv_B_Stat : Terminator
  HeadLampLoFlOn_B_Stat : Terminator
  HeadLampLoFrOn_B_Stat : Terminator
  HeadLampLoOut_B_Stat : Terminator
  HeadLghtHiFdbck_D_Stat : Terminator
  HeadLghtHiOn_B_Stat : Terminator
  HeadLghtSwtch_D_Stat : Terminator
  Headlamp_On_Wrning_Cmd : Terminator
  HomeSafeLtChime_B_Rq : Terminator
  Illuminated_Entry_Stat : Terminator
  ImpactEvntFdbck_D_Stat : Terminator
  KeyInIgnWarn_B_Cmd : Terminator
  Park_Brake_Chime_Rqst : Terminator
  PerimeterAlarmChimeRq : Terminator
  Perimeter_Alarm_Status : Terminator
  PrkLght_D_Stat : Terminator
  PrkLightChime_B_Rq : Terminator
  PudLampDrv_D_Rq : Terminator
  PudLampPsngr_D_Rq : Terminator
  PudLamp_D_Rq : Terminator
  ReducedGuard_D_Stat : Terminator
  RvrseLghtOn_B_Stat : Terminator
  StopLghtOn_B_Stat : Terminator
  TrnNotInPrkChime_B_Rq : Terminator
  WndwGlbl_D_Cmd : Terminator
  WrlssAcsyChrgInhbt_B_Rq : Terminator
  bus_selector : BusSelector  OutputSignals=BrkWarnInd_B_Rq,Brk_Fluid_Lvl_Low,Courtesy_BSave_Stat,Courtesy_Delay_Status,CrnrLghtLeft_Pc_Rq,CrnrLghtRight_Pc_Rq,DayRnngLampOn_B_Stat,DrTgateLck_D_Stat,Dr_Courtesy_Light_Stat,HeadLampLoActv_B_Stat,HeadLampLoFlOn_B_Stat,HeadLampLoFrOn_B_Stat,HeadLampLoOut_B_Stat,HeadLghtHiFdbck_D_Stat,HeadLghtHiOn_B_Stat,HeadLghtSwtch_D_Stat,Headlamp_On_Wrning_Cmd,HomeSafeLtChime_B_Rq,Illuminated_Entry_Stat,ImpactEvntFdbck_D_Stat,KeyInIgnWarn_B_Cmd,Park_Brake_Chime_Rqst,PerimeterAlarmChimeRq,Perimeter_Alarm_Status,PrkLght_D_Stat,PrkLightChime_B_Rq,PudLampDrv_D_Rq,PudLampPsngr_D_Rq,PudLamp_D_Rq,ReducedGuard_D_Stat,RvrseLghtOn_B_Stat,StopLghtOn_B_Stat,TrnNotInPrkChime_B_Rq,WndwGlbl_D_Cmd,WrlssAcsyChrgInhbt_B_Rq
  wires:
  in_port/1 -> bus_selector/1  "BCM_Lamp_Stat_FD1_Ox3C3"
  bus_selector/1 -> BrkWarnInd_B_Rq/1  "<BrkWarnInd_B_Rq>"
  bus_selector/2 -> Brk_Fluid_Lvl_Low/1  "<Brk_Fluid_Lvl_Low>"
  bus_selector/3 -> Courtesy_BSave_Stat/1  "<Courtesy_BSave_Stat>"
  bus_selector/4 -> Courtesy_Delay_Status/1  "<Courtesy_Delay_Status>"
  bus_selector/5 -> CrnrLghtLeft_Pc_Rq/1  "<CrnrLghtLeft_Pc_Rq>"
  bus_selector/6 -> CrnrLghtRight_Pc_Rq/1  "<CrnrLghtRight_Pc_Rq>"
  bus_selector/7 -> DayRnngLampOn_B_Stat/1  "<DayRnngLampOn_B_Stat>"
  bus_selector/8 -> DrTgateLck_D_Stat/1  "<DrTgateLck_D_Stat>"
  bus_selector/9 -> Dr_Courtesy_Light_Stat/1  "<Dr_Courtesy_Light_Stat>"
  bus_selector/10 -> HeadLampLoActv_B_Stat/1  "<HeadLampLoActv_B_Stat>"
  bus_selector/11 -> HeadLampLoFlOn_B_Stat/1  "<HeadLampLoFlOn_B_Stat>"
  bus_selector/12 -> HeadLampLoFrOn_B_Stat/1  "<HeadLampLoFrOn_B_Stat>"
  bus_selector/13 -> HeadLampLoOut_B_Stat/1  "<HeadLampLoOut_B_Stat>"
  bus_selector/14 -> HeadLghtHiFdbck_D_Stat/1  "<HeadLghtHiFdbck_D_Stat>"
  bus_selector/15 -> HeadLghtHiOn_B_Stat/1  "<HeadLghtHiOn_B_Stat>"
  bus_selector/16 -> HeadLghtSwtch_D_Stat/1  "<HeadLghtSwtch_D_Stat>"
  bus_selector/17 -> Headlamp_On_Wrning_Cmd/1  "<Headlamp_On_Wrning_Cmd>"
  bus_selector/18 -> HomeSafeLtChime_B_Rq/1  "<HomeSafeLtChime_B_Rq>"
  bus_selector/19 -> Illuminated_Entry_Stat/1  "<Illuminated_Entry_Stat>"
  bus_selector/20 -> ImpactEvntFdbck_D_Stat/1  "<ImpactEvntFdbck_D_Stat>"
  bus_selector/21 -> KeyInIgnWarn_B_Cmd/1  "<KeyInIgnWarn_B_Cmd>"
  bus_selector/22 -> Park_Brake_Chime_Rqst/1  "<Park_Brake_Chime_Rqst>"
  bus_selector/23 -> PerimeterAlarmChimeRq/1  "<PerimeterAlarmChimeRq>"
  bus_selector/24 -> Perimeter_Alarm_Status/1  "<Perimeter_Alarm_Status>"
  bus_selector/25 -> PrkLght_D_Stat/1  "<PrkLght_D_Stat>"
  bus_selector/26 -> PrkLightChime_B_Rq/1  "<PrkLightChime_B_Rq>"
  bus_selector/27 -> PudLampDrv_D_Rq/1  "<PudLampDrv_D_Rq>"
  bus_selector/28 -> PudLampPsngr_D_Rq/1  "<PudLampPsngr_D_Rq>"
  bus_selector/29 -> PudLamp_D_Rq/1  "<PudLamp_D_Rq>"
  bus_selector/30 -> ReducedGuard_D_Stat/1  "<ReducedGuard_D_Stat>"
  bus_selector/31 -> RvrseLghtOn_B_Stat/1  "<RvrseLghtOn_B_Stat>"
  bus_selector/32 -> StopLghtOn_B_Stat/1  "<StopLghtOn_B_Stat>"
  bus_selector/33 -> TrnNotInPrkChime_B_Rq/1  "<TrnNotInPrkChime_B_Rq>"
  bus_selector/34 -> WndwGlbl_D_Cmd/1  "<WndwGlbl_D_Cmd>"
  bus_selector/35 -> WrlssAcsyChrgInhbt_B_Rq/1  "<WrlssAcsyChrgInhbt_B_Rq>"

== system test_mdl_NI/Subsystem/GWM/BattRgenLo_1_FD1_Ox361 ==
  in_port : Inport
  BattRgenLo_I_Actl : Terminator
  BattRgenLo_U_Actl : Terminator
  bus_selector : BusSelector  OutputSignals=BattRgenLo_I_Actl,BattRgenLo_U_Actl
  wires:
  in_port/1 -> bus_selector/1  "BattRgenLo_1_FD1_Ox361"
  bus_selector/1 -> BattRgenLo_I_Actl/1  "<BattRgenLo_I_Actl>"
  bus_selector/2 -> BattRgenLo_U_Actl/1  "<BattRgenLo_U_Actl>"

== system test_mdl_NI/Subsystem/GWM/BattRgenLo_2_FD1_Ox362 ==
  in_port : Inport
  BattRgenLoChrg_I_Mx : Terminator
  BattRgenLoChrg_U_Mx : Terminator
  BattRgenLoDchrg_I_Mx : Terminator
  BattRgenLoDchrg_U_Mn : Terminator
  BattRgenLoOpen_U_Actl : Terminator
  bus_selector : BusSelector  OutputSignals=BattRgenLoChrg_I_Mx,BattRgenLoChrg_U_Mx,BattRgenLoDchrg_I_Mx,BattRgenLoDchrg_U_Mn,BattRgenLoOpen_U_Actl
  wires:
  in_port/1 -> bus_selector/1  "BattRgenLo_2_FD1_Ox362"
  bus_selector/1 -> BattRgenLoChrg_I_Mx/1  "<BattRgenLoChrg_I_Mx>"
  bus_selector/2 -> BattRgenLoChrg_U_Mx/1  "<BattRgenLoChrg_U_Mx>"
  bus_selector/3 -> BattRgenLoDchrg_I_Mx/1  "<BattRgenLoDchrg_I_Mx>"
  bus_selector/4 -> BattRgenLoDchrg_U_Mn/1  "<BattRgenLoDchrg_U_Mn>"
  bus_selector/5 -> BattRgenLoOpen_U_Actl/1  "<BattRgenLoOpen_U_Actl>"

== system test_mdl_NI/Subsystem/GWM/BattRgenLo_3_FD1_Ox363 ==
  in_port : Inport
  BattRgenLoBalnc_B_Rq : Terminator
  BattRgenLo_AhRide_Actl : Terminator
  BattRgenLo_Ah_Actl : Terminator
  BattRgenLo_R_Actl : Terminator
  BattRgenLo_Te_Actl : Terminator
  BattRgenLo_Te_Hi : Terminator
  bus_selector : BusSelector  OutputSignals=BattRgenLoBalnc_B_Rq,BattRgenLo_AhRide_Actl,BattRgenLo_Ah_Actl,BattRgenLo_R_Actl,BattRgenLo_Te_Actl,BattRgenLo_Te_Hi
  wires:
  in_port/1 -> bus_selector/1  "BattRgenLo_3_FD1_Ox363"
  bus_selector/1 -> BattRgenLoBalnc_B_Rq/1  "<BattRgenLoBalnc_B_Rq>"
  bus_selector/2 -> BattRgenLo_AhRide_Actl/1  "<BattRgenLo_AhRide_Actl>"
  bus_selector/3 -> BattRgenLo_Ah_Actl/1  "<BattRgenLo_Ah_Actl>"
  bus_selector/4 -> BattRgenLo_R_Actl/1  "<BattRgenLo_R_Actl>"
  bus_selector/5 -> BattRgenLo_Te_Actl/1  "<BattRgenLo_Te_Actl>"
  bus_selector/6 -> BattRgenLo_Te_Hi/1  "<BattRgenLo_Te_Hi>"

== system test_mdl_NI/Subsystem/GWM/BattRgenLo_4_FD1_Ox364 ==
  in_port : Inport
  BattRgenLoChrg_B_Rq : Terminator
  BattRgenLoChrg_D_Stat : Terminator
  BattRgenLoDChrg_D_Stat : Terminator
  BattRgenLoDchrg_B_Rq : Terminator
  BattRgenLoPrtct_B_Stat : Terminator
  BattRgenLoPulse_U_Pred : Terminator
  BattRgenLoSoc_Pc_Actl : Terminator
  BattRgenLoStat_D_Qlty : Terminator
  BattRgenLo_B_Falt : Terminator
  BattRgenLo_T_Est : Terminator
  bus_selector : BusSelector  OutputSignals=BattRgenLoChrg_B_Rq,BattRgenLoChrg_D_Stat,BattRgenLoDChrg_D_Stat,BattRgenLoDchrg_B_Rq,BattRgenLoPrtct_B_Stat,BattRgenLoPulse_U_Pred,BattRgenLoSoc_Pc_Actl,BattRgenLoStat_D_Qlty,BattRgenLo_B_Falt,BattRgenLo_T_Est
  wires:
  in_port/1 -> bus_selector/1  "BattRgenLo_4_FD1_Ox364"
  bus_selector/1 -> BattRgenLoChrg_B_Rq/1  "<BattRgenLoChrg_B_Rq>"
  bus_selector/2 -> BattRgenLoChrg_D_Stat/1  "<BattRgenLoChrg_D_Stat>"
  bus_selector/3 -> BattRgenLoDChrg_D_Stat/1  "<BattRgenLoDChrg_D_Stat>"
  bus_selector/4 -> BattRgenLoDchrg_B_Rq/1  "<BattRgenLoDchrg_B_Rq>"
  bus_selector/5 -> BattRgenLoPrtct_B_Stat/1  "<BattRgenLoPrtct_B_Stat>"
  bus_selector/6 -> BattRgenLoPulse_U_Pred/1  "<BattRgenLoPulse_U_Pred>"
  bus_selector/7 -> BattRgenLoSoc_Pc_Actl/1  "<BattRgenLoSoc_Pc_Actl>"
  bus_selector/8 -> BattRgenLoStat_D_Qlty/1  "<BattRgenLoStat_D_Qlty>"
  bus_selector/9 -> BattRgenLo_B_Falt/1  "<BattRgenLo_B_Falt>"
  bus_selector/10 -> BattRgenLo_T_Est/1  "<BattRgenLo_T_Est>"

== system test_mdl_NI/Subsystem/GWM/Battery_Mgmt_24V_FD1_Ox42E ==
  in_port : Inport
  BattULo24Soc_Pc_Actl : Terminator
  BattULo24State_D_Qlty : Terminator
  BattULo24_Ah_DeltaRide : Terminator
  BattULo24_B_Falt : Terminator
  BattULo24_D_Falt : Terminator
  BattULo24_I_Actl : Terminator
  BattULo24_Te_Actl : Terminator
  bus_selector : BusSelector  OutputSignals=BattULo24Soc_Pc_Actl,BattULo24State_D_Qlty,BattULo24_Ah_DeltaRide,BattULo24_B_Falt,BattULo24_D_Falt,BattULo24_I_Actl,BattULo24_Te_Actl
  wires:
  in_port/1 -> bus_selector/1  "Battery_Mgmt_24V_FD1_Ox42E"
  bus_selector/1 -> BattULo24Soc_Pc_Actl/1  "<BattULo24Soc_Pc_Actl>"
  bus_selector/2 -> BattULo24State_D_Qlty/1  "<BattULo24State_D_Qlty>"
  bus_selector/3 -> BattULo24_Ah_DeltaRide/1  "<BattULo24_Ah_DeltaRide>"
  bus_selector/4 -> BattULo24_B_Falt/1  "<BattULo24_B_Falt>"
  bus_selector/5 -> BattULo24_D_Falt/1  "<BattULo24_D_Falt>"
  bus_selector/6 -> BattULo24_I_Actl/1  "<BattULo24_I_Actl>"
  bus_selector/7 -> BattULo24_Te_Actl/1  "<BattULo24_Te_Actl>"

== system test_mdl_NI/Subsystem/GWM/Battery_Mgmt_2_FD1_Ox42C ==
  in_port : Inport
  BattULoChrg_D_Rq : Terminator
  BattULoSrvc_T_Actl : Terminator
  Batt_Crit_SoC_B : Terminator
  Batt_Lo_SoC_B : Terminator
  ChargeMode : Terminator
  EngStrtInhbt_B_RqBatt : Terminator
  IdleSpeedIncrease_El : Terminator
  PeriodicElLoad_B_Stat : Terminator
  PwSysULoFalt_D_Stat : Terminator
  Shed_Drain_Eng_Off_B : Terminator
  Shed_Feature_Group_ID : Terminator
  Shed_Level_Req : Terminator
  Shed_T_Eng_Off_B : Terminator
  ULoRgenTestMde_B_Rq : Terminator
  bus_selector : BusSelector  OutputSignals=BattULoChrg_D_Rq,BattULoSrvc_T_Actl,Batt_Crit_SoC_B,Batt_Lo_SoC_B,ChargeMode,EngStrtInhbt_B_RqBatt,IdleSpeedIncrease_El,PeriodicElLoad_B_Stat,PwSysULoFalt_D_Stat,Shed_Drain_Eng_Off_B,Shed_Feature_Group_ID,Shed_Level_Req,Shed_T_Eng_Off_B,ULoRgenTestMde_B_Rq
  wires:
  in_port/1 -> bus_selector/1  "Battery_Mgmt_2_FD1_Ox42C"
  bus_selector/1 -> BattULoChrg_D_Rq/1  "<BattULoChrg_D_Rq>"
  bus_selector/2 -> BattULoSrvc_T_Actl/1  "<BattULoSrvc_T_Actl>"
  bus_selector/3 -> Batt_Crit_SoC_B/1  "<Batt_Crit_SoC_B>"
  bus_selector/4 -> Batt_Lo_SoC_B/1  "<Batt_Lo_SoC_B>"
  bus_selector/5 -> ChargeMode/1  "<ChargeMode>"
  bus_selector/6 -> EngStrtInhbt_B_RqBatt/1  "<EngStrtInhbt_B_RqBatt>"
  bus_selector/7 -> IdleSpeedIncrease_El/1  "<IdleSpeedIncrease_El>"
  bus_selector/8 -> PeriodicElLoad_B_Stat/1  "<PeriodicElLoad_B_Stat>"
  bus_selector/9 -> PwSysULoFalt_D_Stat/1  "<PwSysULoFalt_D_Stat>"
  bus_selector/10 -> Shed_Drain_Eng_Off_B/1  "<Shed_Drain_Eng_Off_B>"
  bus_selector/11 -> Shed_Feature_Group_ID/1  "<Shed_Feature_Group_ID>"
  bus_selector/12 -> Shed_Level_Req/1  "<Shed_Level_Req>"
  bus_selector/13 -> Shed_T_Eng_Off_B/1  "<Shed_T_Eng_Off_B>"
  bus_selector/14 -> ULoRgenTestMde_B_Rq/1  "<ULoRgenTestMde_B_Rq>"

== system test_mdl_NI/Subsystem/GWM/Battery_Mgmt_3_FD1_Ox43C ==
  in_port : Inport
  BSBattQCapAh : Terminator
  BSBattQDeltaRideAh : Terminator
  BSBattSOC : Terminator
  BSFault : Terminator
  BattULo2_Te_Actl : Terminator
  BattULoChrg_URate_RqMx : Terminator
  BattULoChrg_U_RqMn : Terminator
  BattULoChrg_U_RqMx : Terminator
  BattULoState_D_Qlty : Terminator
  bus_selector : BusSelector  OutputSignals=BSBattQCapAh,BSBattQDeltaRideAh,BSBattSOC,BSFault,BattULo2_Te_Actl,BattULoChrg_URate_RqMx,BattULoChrg_U_RqMn,BattULoChrg_U_RqMx,BattULoState_D_Qlty
  wires:
  in_port/1 -> bus_selector/1  "Battery_Mgmt_3_FD1_Ox43C"
  bus_selector/1 -> BSBattQCapAh/1  "<BSBattQCapAh>"
  bus_selector/2 -> BSBattQDeltaRideAh/1  "<BSBattQDeltaRideAh>"
  bus_selector/3 -> BSBattSOC/1  "<BSBattSOC>"
  bus_selector/4 -> BSFault/1  "<BSFault>"
  bus_selector/5 -> BattULo2_Te_Actl/1  "<BattULo2_Te_Actl>"
  bus_selector/6 -> BattULoChrg_URate_RqMx/1  "<BattULoChrg_URate_RqMx>"
  bus_selector/7 -> BattULoChrg_U_RqMn/1  "<BattULoChrg_U_RqMn>"
  bus_selector/8 -> BattULoChrg_U_RqMx/1  "<BattULoChrg_U_RqMx>"
  bus_selector/9 -> BattULoState_D_Qlty/1  "<BattULoState_D_Qlty>"

== system test_mdl_NI/Subsystem/GWM/Battery_Mgmt_4_FD1_Ox42B ==
  in_port : Inport
  BattULoAuxIsol_D_Rq : Terminator
  BattULoAuxSoc_Pc_Actl : Terminator
  BattULoAux_B_Falt : Terminator
  BattULoAux_D_Qlty : Terminator
  BattULoAux_I_Actl : Terminator
  BattULoAux_U_Actl : Terminator
  BattULoAux_U_Rq : Terminator
  BattULoCrnkBelt_U_Pred : Terminator
  BattULoCrnkStrt_U_Pred : Terminator
  bus_selector : BusSelector  OutputSignals=BattULoAuxIsol_D_Rq,BattULoAuxSoc_Pc_Actl,BattULoAux_B_Falt,BattULoAux_D_Qlty,BattULoAux_I_Actl,BattULoAux_U_Actl,BattULoAux_U_Rq,BattULoCrnkBelt_U_Pred,BattULoCrnkStrt_U_Pred
  wires:
  in_port/1 -> bus_selector/1  "Battery_Mgmt_4_FD1_Ox42B"
  bus_selector/1 -> BattULoAuxIsol_D_Rq/1  "<BattULoAuxIsol_D_Rq>"
  bus_selector/2 -> BattULoAuxSoc_Pc_Actl/1  "<BattULoAuxSoc_Pc_Actl>"
  bus_selector/3 -> BattULoAux_B_Falt/1  "<BattULoAux_B_Falt>"
  bus_selector/4 -> BattULoAux_D_Qlty/1  "<BattULoAux_D_Qlty>"
  bus_selector/5 -> BattULoAux_I_Actl/1  "<BattULoAux_I_Actl>"
  bus_selector/6 -> BattULoAux_U_Actl/1  "<BattULoAux_U_Actl>"
  bus_selector/7 -> BattULoAux_U_Rq/1  "<BattULoAux_U_Rq>"
  bus_selector/8 -> BattULoCrnkBelt_U_Pred/1  "<BattULoCrnkBelt_U_Pred>"
  bus_selector/9 -> BattULoCrnkStrt_U_Pred/1  "<BattULoCrnkStrt_U_Pred>"

== system test_mdl_NI/Subsystem/GWM/Battery_Traction_1_FD1_Ox7A ==
  in_port : Inport
  BattTracMil_D_Rq : Terminator
  BattTracOffFst_D_Actl : Terminator
  BattTracOff_B_Actl : Terminator
  BattTrac_I_Actl : Terminator
  BattTrac_U_Actl : Terminator
  BattTrac_U_LimHi : Terminator
  BattTrac_U_LimLo : Terminator
  VehStrtInhbt_B_RqBatt : Terminator
  bus_selector : BusSelector  OutputSignals=BattTracMil_D_Rq,BattTracOffFst_D_Actl,BattTracOff_B_Actl,BattTrac_I_Actl,BattTrac_U_Actl,BattTrac_U_LimHi,BattTrac_U_LimLo,VehStrtInhbt_B_RqBatt
  wires:
  in_port/1 -> bus_selector/1  "Battery_Traction_1_FD1_Ox7A"
  bus_selector/1 -> BattTracMil_D_Rq/1  "<BattTracMil_D_Rq>"
  bus_selector/2 -> BattTracOffFst_D_Actl/1  "<BattTracOffFst_D_Actl>"
  bus_selector/3 -> BattTracOff_B_Actl/1  "<BattTracOff_B_Actl>"
  bus_selector/4 -> BattTrac_I_Actl/1  "<BattTrac_I_Actl>"
  bus_selector/5 -> BattTrac_U_Actl/1  "<BattTrac_U_Actl>"
  bus_selector/6 -> BattTrac_U_LimHi/1  "<BattTrac_U_LimHi>"
  bus_selector/7 -> BattTrac_U_LimLo/1  "<BattTrac_U_LimLo>"
  bus_selector/8 -> VehStrtInhbt_B_RqBatt/1  "<VehStrtInhbt_B_RqBatt>"

== system test_mdl_NI/Subsystem/GWM/Battery_Traction_3_FD1_Ox24B ==
  in_port : Inport
  BattTracClnt_Te_Actl : Terminator
  BattTracSoc_Pc_LimHi : Terminator
  BattTracSoc_Pc_LimLo : Terminator
  BattTracSoc_Pc_MnPrtct : Terminator
  BattTracSoc_Pc_MxPrtct : Terminator
  BattTracSrvcRqd_B_Rq : Terminator
  BattTracWarnLamp_B_Rq : Terminator
  bus_selector : BusSelector  OutputSignals=BattTracClnt_Te_Actl,BattTracSoc_Pc_LimHi,BattTracSoc_Pc_LimLo,BattTracSoc_Pc_MnPrtct,BattTracSoc_Pc_MxPrtct,BattTracSrvcRqd_B_Rq,BattTracWarnLamp_B_Rq
  wires:
  in_port/1 -> bus_selector/1  "Battery_Traction_3_FD1_Ox24B"
  bus_selector/1 -> BattTracClnt_Te_Actl/1  "<BattTracClnt_Te_Actl>"
  bus_selector/2 -> BattTracSoc_Pc_LimHi/1  "<BattTracSoc_Pc_LimHi>"
  bus_selector/3 -> BattTracSoc_Pc_LimLo/1  "<BattTracSoc_Pc_LimLo>"
  bus_selector/4 -> BattTracSoc_Pc_MnPrtct/1  "<BattTracSoc_Pc_MnPrtct>"
  bus_selector/5 -> BattTracSoc_Pc_MxPrtct/1  "<BattTracSoc_Pc_MxPrtct>"
  bus_selector/6 -> BattTracSrvcRqd_B_Rq/1  "<BattTracSrvcRqd_B_Rq>"
  bus_selector/7 -> BattTracWarnLamp_B_Rq/1  "<BattTracWarnLamp_B_Rq>"

== system test_mdl_NI/Subsystem/GWM/Battery_Traction_4_FD1_Ox24C ==
  in_port : Inport
  BattTracDiagClr_B_Rq : Terminator
  BattTracSoc2_Pc_Actl : Terminator
  BattTrac_Te_Actl : Terminator
  bus_selector : BusSelector  OutputSignals=BattTracDiagClr_B_Rq,BattTracSoc2_Pc_Actl,BattTrac_Te_Actl
  wires:
  in_port/1 -> bus_selector/1  "Battery_Traction_4_FD1_Ox24C"
  bus_selector/1 -> BattTracDiagClr_B_Rq/1  "<BattTracDiagClr_B_Rq>"
  bus_selector/2 -> BattTracSoc2_Pc_Actl/1  "<BattTracSoc2_Pc_Actl>"
  bus_selector/3 -> BattTrac_Te_Actl/1  "<BattTrac_Te_Actl>"

== system test_mdl_NI/Subsystem/GWM/Battery_Traction_5_FD1_Ox24D ==
  in_port : Inport
  BattTrac2_Pw_ChrgInst : Terminator
  BattTrac2_Pw_DchrgInst : Terminator
  BattTrac2_Pw_LimChrg : Terminator
  BattTrac2_Pw_LimDchrg : Terminator
  bus_selector : BusSelector  OutputSignals=BattTrac2_Pw_ChrgInst,BattTrac2_Pw_DchrgInst,BattTrac2_Pw_LimChrg,BattTrac2_Pw_LimDchrg
  wires:
  in_port/1 -> bus_selector/1  "Battery_Traction_5_FD1_Ox24D"
  bus_selector/1 -> BattTrac2_Pw_ChrgInst/1  "<BattTrac2_Pw_ChrgInst>"
  bus_selector/2 -> BattTrac2_Pw_DchrgInst/1  "<BattTrac2_Pw_DchrgInst>"
  bus_selector/3 -> BattTrac2_Pw_LimChrg/1  "<BattTrac2_Pw_LimChrg>"
  bus_selector/4 -> BattTrac2_Pw_LimDchrg/1  "<BattTrac2_Pw_LimDchrg>"

== system test_mdl_NI/Subsystem/GWM/Battery_Traction_6_FD1_Ox458 ==
  in_port : Inport
  BattTracChrgSustn_B_Rq : Terminator
  BattTracClntPmp_D_Stat : Terminator
  BattTracCnnct_D_Cmd : Terminator
  BattTracDcdcDis_B_Rq : Terminator
  BattTracDelta_Te_Actl : Terminator
  BattTracHvilOpen_B_Stat : Terminator
  HtrnClntPump_D_Stat : Terminator
  bus_selector : BusSelector  OutputSignals=BattTracChrgSustn_B_Rq,BattTracClntPmp_D_Stat,BattTracCnnct_D_Cmd,BattTracDcdcDis_B_Rq,BattTracDelta_Te_Actl,BattTracHvilOpen_B_Stat,HtrnClntPump_D_Stat
  wires:
  in_port/1 -> bus_selector/1  "Battery_Traction_6_FD1_Ox458"
  bus_selector/1 -> BattTracChrgSustn_B_Rq/1  "<BattTracChrgSustn_B_Rq>"
  bus_selector/2 -> BattTracClntPmp_D_Stat/1  "<BattTracClntPmp_D_Stat>"
  bus_selector/3 -> BattTracCnnct_D_Cmd/1  "<BattTracCnnct_D_Cmd>"
  bus_selector/4 -> BattTracDcdcDis_B_Rq/1  "<BattTracDcdcDis_B_Rq>"
  bus_selector/5 -> BattTracDelta_Te_Actl/1  "<BattTracDelta_Te_Actl>"
  bus_selector/6 -> BattTracHvilOpen_B_Stat/1  "<BattTracHvilOpen_B_Stat>"
  bus_selector/7 -> HtrnClntPump_D_Stat/1  "<HtrnClntPump_D_Stat>"

== system test_mdl_NI/Subsystem/GWM/BodyInfo_3_FD1_Ox3B3 ==
  in_port : Inport
  Backlit_LED_Status : Terminator
  BodySrvcRqd_B_Rq : Terminator
  CrashEvnt_D_Stat : Terminator
  Day_Night_Status : Terminator
  Delay_Accy : Terminator
  DimmingLvlEvnt_No_Actl : Terminator
  Dimming_Lvl : Terminator
  DrStatDrvErrCnt_B_Stat : Terminator
  DrStatDrv_B_Actl : Terminator
  DrStatHood_B_Actl : Terminator
  DrStatInnrTgate_B_Actl : Terminator
  DrStatPsngr_B_Actl : Terminator
  DrStatRl_B_Actl : Terminator
  DrStatRr_B_Actl : Terminator
  DrStatTgate_B_Actl : Terminator
  FogLghtFrontOn_B_Stat : Terminator
  FogLghtRearOn_B_Stat : Terminator
  FuelPmpInhbt_B_Stat : Terminator
  IgnKeyType_D_Actl : Terminator
  Ignition_Status : Terminator
  Key_In_Ignition_Stat : Terminator
  LifeCycMde_D_Actl : Terminator
  Litval : Terminator
  Parklamp_Status : Terminator
  PrkBrkActv_B_Actl : Terminator
  Remote_Start_Status : Terminator
  TurnLghtLeftOn_B_Stat : Terminator
  TurnLghtLeft_D_Rq : Terminator
  TurnLghtRightOn_B_Stat : Terminator
  TurnLghtRight_D_Rq : Terminator
  ValetMode_D_Mem : Terminator
  bus_selector : BusSelector  OutputSignals=Backlit_LED_Status,BodySrvcRqd_B_Rq,CrashEvnt_D_Stat,Day_Night_Status,Delay_Accy,DimmingLvlEvnt_No_Actl,Dimming_Lvl,DrStatDrvErrCnt_B_Stat,DrStatDrv_B_Actl,DrStatHood_B_Actl,DrStatInnrTgate_B_Actl,DrStatPsngr_B_Actl,DrStatRl_B_Actl,DrStatRr_B_Actl,DrStatTgate_B_Actl,FogLghtFrontOn_B_Stat,FogLghtRearOn_B_Stat,FuelPmpInhbt_B_Stat,IgnKeyType_D_Actl,Ignition_Status,Key_In_Ignition_Stat,LifeCycMde_D_Actl,Litval,Parklamp_Status,PrkBrkActv_B_Actl,Remote_Start_Status,TurnLghtLeftOn_B_Stat,TurnLghtLeft_D_Rq,TurnLghtRightOn_B_Stat,TurnLghtRight_D_Rq,ValetMode_D_Mem
  wires:
  in_port/1 -> bus_selector/1  "BodyInfo_3_FD1_Ox3B3"
  bus_selector/1 -> Backlit_LED_Status/1  "<Backlit_LED_Status>"
  bus_selector/2 -> BodySrvcRqd_B_Rq/1  "<BodySrvcRqd_B_Rq>"
  bus_selector/3 -> CrashEvnt_D_Stat/1  "<CrashEvnt_D_Stat>"
  bus_selector/4 -> Day_Night_Status/1  "<Day_Night_Status>"
  bus_selector/5 -> Delay_Accy/1  "<Delay_Accy>"
  bus_selector/6 -> DimmingLvlEvnt_No_Actl/1  "<DimmingLvlEvnt_No_Actl>"
  bus_selector/7 -> Dimming_Lvl/1  "<Dimming_Lvl>"
  bus_selector/8 -> DrStatDrvErrCnt_B_Stat/1  "<DrStatDrvErrCnt_B_Stat>"
  bus_selector/9 -> DrStatDrv_B_Actl/1  "<DrStatDrv_B_Actl>"
  bus_selector/10 -> DrStatHood_B_Actl/1  "<DrStatHood_B_Actl>"
  bus_selector/11 -> DrStatInnrTgate_B_Actl/1  "<DrStatInnrTgate_B_Actl>"
  bus_selector/12 -> DrStatPsngr_B_Actl/1  "<DrStatPsngr_B_Actl>"
  bus_selector/13 -> DrStatRl_B_Actl/1  "<DrStatRl_B_Actl>"
  bus_selector/14 -> DrStatRr_B_Actl/1  "<DrStatRr_B_Actl>"
  bus_selector/15 -> DrStatTgate_B_Actl/1  "<DrStatTgate_B_Actl>"
  bus_selector/16 -> FogLghtFrontOn_B_Stat/1  "<FogLghtFrontOn_B_Stat>"
  bus_selector/17 -> FogLghtRearOn_B_Stat/1  "<FogLghtRearOn_B_Stat>"
  bus_selector/18 -> FuelPmpInhbt_B_Stat/1  "<FuelPmpInhbt_B_Stat>"
  bus_selector/19 -> IgnKeyType_D_Actl/1  "<IgnKeyType_D_Actl>"
  bus_selector/20 -> Ignition_Status/1  "<Ignition_Status>"
  bus_selector/21 -> Key_In_Ignition_Stat/1  "<Key_In_Ignition_Stat>"
  bus_selector/22 -> LifeCycMde_D_Actl/1  "<LifeCycMde_D_Actl>"
  bus_selector/23 -> Litval/1  "<Litval>"
  bus_selector/24 -> Parklamp_Status/1  "<Parklamp_Status>"
  bus_selector/25 -> PrkBrkActv_B_Actl/1  "<PrkBrkActv_B_Actl>"
  bus_selector/26 -> Remote_Start_Status/1  "<Remote_Start_Status>"
  bus_selector/27 -> TurnLghtLeftOn_B_Stat/1  "<TurnLghtLeftOn_B_Stat>"
  bus_selector/28 -> TurnLghtLeft_D_Rq/1  "<TurnLghtLeft_D_Rq>"
  bus_selector/29 -> TurnLghtRightOn_B_Stat/1  "<TurnLghtRightOn_B_Stat>"
  bus_selector/30 -> TurnLghtRight_D_Rq/1  "<TurnLghtRight_D_Rq>"
  bus_selector/31 -> ValetMode_D_Mem/1  "<ValetMode_D_Mem>"

== system test_mdl_NI/Subsystem/GWM/Body_Info_10_FD1_Ox3BA ==
  in_port : Inport
  GenericSwtch1_No_Actl : Terminator
  GenericSwtch2_No_Actl : Terminator
  GenericSwtch3_No_Actl : Terminator
  bus_selector : BusSelector  OutputSignals=GenericSwtch1_No_Actl,GenericSwtch2_No_Actl,GenericSwtch3_No_Actl
  wires:
  in_port/1 -> bus_selector/1  "Body_Info_10_FD1_Ox3BA"
  bus_selector/1 -> GenericSwtch1_No_Actl/1  "<GenericSwtch1_No_Actl>"
  bus_selector/2 -> GenericSwtch2_No_Actl/1  "<GenericSwtch2_No_Actl>"
  bus_selector/3 -> GenericSwtch3_No_Actl/1  "<GenericSwtch3_No_Actl>"
